simulink model "I2C_V2"  (R2017b)
settings: Solver=FixedStepAuto  StartTime=0.0  StopTime=10.0  RelTol=1e-3
PreLoadFcn:
  | waijung.modelPreload; % Required for working with Waijung Blockset. Do not remove.
undefined symbols (not defined in the file): HSEOSC, Link, LQFP100, ST, STM32F407VG
libraries: simulink x51, stm32f4_i2c_lib x7, stm32f4_io_lib x2, stm32f4_device_config_lib x1
(part 1 of 2)
CloseFcn:
  | waijung.modelClose; % Required for working with Waijung Blockset. Do not remove.
settings Model: Creator=Sputnik  LastModifiedBy=Sputnik
settings OptimizationCC: DefaultParameterBehavior=Inlined  PassReuseOutputArgsAs=Individual arguments
settings DebuggingCC: ParameterTunabilityLossMsg=error
settings HardwareCC: ProdBitPerPointer=32  ProdBitPerSizeT=32  ProdBitPerPtrDiffT=32  ProdLargestAtomicFloat=None  ProdIntDivRoundTo=Undefined  ProdWordSize=32  ProdHWDeviceType=ARM Compatible->Cortex - M4  TargetEndianess=LittleEndian  TargetHWDeviceType=ARM Compatible->Cortex - M4
settings SFSimCC: MATLABDynamicMemAlloc=off
settings RTWCC: SystemTargetFile=stm32f4.tlc  GenerateMakefile=off  TemplateMakefile=ert_default_tmf  Description=STM32F4 Target  GenerateReport=on  IncludeHyperlinkInReport=on  LaunchReport=on  GenerateTraceInfo=on  GenerateTraceReport=on  GenerateTraceReportSl=on  GenerateTraceReportSf=on  GenerateTraceReportEml=on
settings CodeAppCC: ForceParamTrailComments=on  IgnoreCustomStorageClasses=off  OperatorAnnotations=on  SimulinkDataObjDesc=on  SFDataObjDesc=on  InsertBlockDesc=on
settings STFCustomTargetCC: TargetLangStandard=C99 (ISO)  MultiwordLength=256  ModelReferenceCompliant=off  CombineOutputUpdateFcns=on  ERTCustomFileBanners=on  SupportContinuousTime=off  SupportNonInlinedSFcns=off  RemoveResetFunc=on  MATLABClassNameForMDSCustomization=Simulink.SoftwareTarget.ERTCustomization  GRTInterface=off  SystemTargetFile=stm32f4.tlc
settings ERTTargetCC: TargetLangStandard=C99 (ISO)  ModelReferenceCompliant=off  ParMdlRefBuildCompliant=off  CompOptLevelCompliant=off  ConcurrentExecutionCompliant=off  ModelStepFunctionPrototypeControlCompliant=off  CPPClassGenCompliant=off  UseToolchainInfoCompliant=off  InlinedParameterPlacement=NonHierarchical  ERTSrcFileBannerTemplate=stm32f4_code_template.cgt  ERTHdrFileBannerTemplate=stm32f4_code_template.cgt  ERTDataSrcFileTemplate=stm32f4_code_template.cgt  ERTDataHdrFileTemplate=stm32f4_code_template.cgt  ERTCustomFileTemplate=stm32f4_file_process.tlc

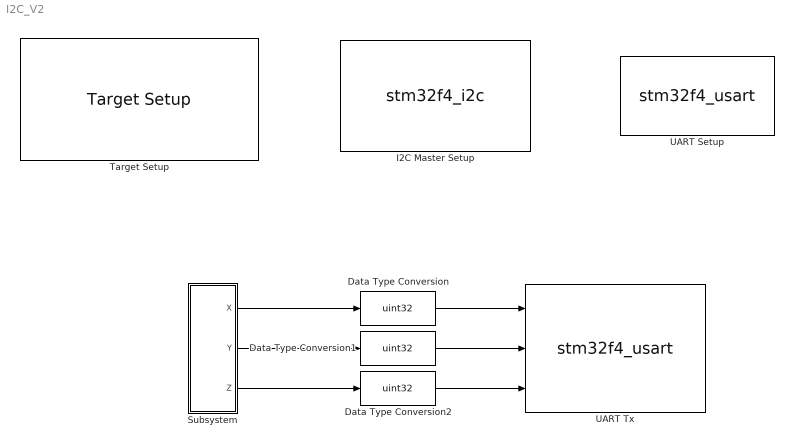
== system I2C_V2 ==
  Data Type Conversion : DataTypeConversion  OutDataTypeStr=uint32
  Data Type Conversion1 : DataTypeConversion  OutDataTypeStr=uint32
  Data Type Conversion2 : DataTypeConversion  OutDataTypeStr=uint32
  I2C Master Setup : S-Function  FunctionName=stm32f4_i2c  Parameters=configuration,module,transfer,clkspeed,timeout,sdapin,sclpin,writecount,readcount,inputtypearray,outputtypearray,confstr,sampletime,sampletimestr,blockid  SFunctionDeploymentMode=off  EnableBusSupport=off  mask(stm32f4_i2c){configuration=Setup, module=1, lastmodule=1, transfer=Blocking, dutycycle=TLow/THigh = 2, clkspeed=400, timeout=25, writecount=0, readcount=0, sdapin=B7, sclpin=B6, waitwritetime=0, inputtypearray=[0], outputtypearray=[0], confstr=["B","7","B","6","1","1","6","0","I2C_DutyCycle_2","0","off"], sampletime=-1, sampletimestr=-1, blockid=I2CMasterSetup}
      mask prompts: module "I2C Module"; lastmodule "Last module"; transfer "Transfer mode"; dutycycle "Duty cycle in fast mode"; clkspeed "Clock speed (kHz)"; timeout "Timeout (ms)"; writecount "Bytes write count"; readcount "Bytes read count"; sdapin "SDA pin"; sclpin "SCL pin"; waitwritetime "Wait write time (ms), default is 0"; inputtypearray "Input type array"; outputtypearray "Output type array"; confstr "Configuration string"; sampletime "Sample time (sec)"; sampletimestr "Compiled sample time (sec) in string"
      mask init:
      | stm32f4_i2c_callback('init');
      mask Help: web(fullfile(waijungdocroot,'stm32f4_i2c_setup.htm'), '-browser')
      mask TypeOptions configuration: Setup | Transaction
      mask Callback configuration: stm32f4_i2c_callback('configuration');
      mask TypeOptions module: 1 | 2 | 3
      mask Callback module: stm32f4_i2c_callback('module');
      mask TypeOptions transfer: Blocking | Non-blocking
      mask TypeOptions dutycycle: TLow/THigh = 16/9 | TLow/THigh = 2
      mask Callback dutycycle: stm32f4_i2c_callback('dutycycle');
      mask Callback writecount: stm32f4_i2c_callback('writecount');
      mask Callback readcount: stm32f4_i2c_callback('readcount');
      mask TypeOptions sdapin: Not used | B7 | B9
      mask Callback sdapin: stm32f4_i2c_callback('sdapin');
      mask TypeOptions sclpin: Not used | B6 | B8
      mask Callback sclpin: stm32f4_i2c_callback('sclpin');
      mask Callback confstr: stm32f4_i2c_callback('confstr');
      mask Callback sampletime: stm32f4_i2c_callback('sampletime');
      mask Callback sampletimestr: stm32f4_i2c_callback('sampletimestr');
      mask Callback blockid: stm32f4_i2c_callback('blockid');
      mask Display: text(0.5, 0.5, 'Module: I2C1\nClock: 400kHz\nSDA/SCL Pin: B7/B6','ver','middle','hor','center');
  Subsystem : Subsystem
  Target Setup : stm32f4_device_config_lib/Target Setup  Priority=100  compiler=GNU ARM  previous_compiler=GNU ARM  mcu=STM32F407VG (LQFP100)  mcustr=STM32F407VG  clockconfig=HSEOSC-8MHz  system_stm32f4xx_c_path=C:\Users\Sputnik\Downloads\waijung17_03a\targets\stm32f4_target\stm32f4\utils\system_stm32f4xx_default\STM32F40_41xxx\hseosc8mhz  showmemoryconfiguration=off  stacksize=0x2000  heapsize=0x2000  enableautocompiledownload=on  fullchiperase=off  programmerinterface=ST-Link  editctrlstr=on  compilercontrolstr=$(patsubst %, -I%, .) -mcpu=cortex-m4 -mthumb -mthumb-interwork -mfloat-abi=hard -mfpu=fpv4-sp-d16 -ffast-math -Wall -Wextra -Ofast  assemblercontrolstr=$(patsubst %, -I%, .) -mcpu=cortex-m4 -mthumb -mthumb-interwork -mfloat-abi=hard -mfpu=fpv4-sp-d16 -ffast-math -Wall -Wextra -Ofast -Wa,-amhls=$(<:.s=.lst) -D__STACK_SIZE=$(STACK_SIZE) -D__HEAP_SIZE=$(HEAP_SIZE)  linkercontrolstr=-T$(LD_SCRIPT) -g -Wl,-Map=$(MAP),--cref,--no-warn-mismatch -mcpu=cortex-m4 -mthumb -mthumb-interwork -mfloat-abi=hard -mfpu=fpv4-sp-d16  runafterdownload=on  execprofile=None  profileruart=3  profilerbaud=500000  profilertxpin=D8  profilerinitstr=0.005,168000000,840000,500000,0  manualsetsampletime=on  sampletime=0.005  blockid=TargetSetup  systickreloadvalue=840000  hseval=8000000  lastprofileruart=3  hclk=168000000  flashorigin=0x8000000  flashlength=1024k  ramorigin=0x20000000  ramlength=128k  useextram=off
      settings: SourceProductName=Waijung Blockset
  UART Setup : S-Function  Priority=1  FunctionName=stm32f4_usart  Parameters=configuration,uartmodule,transfer,baudrate,inputtype,outputtype,confstr,binheaderarray,binterminatorarray,asciiheader,asciiterminator,bindatalength,packetmode,varname,sampletime,sampletimestr,blockid  SFunctionDeploymentMode=off  EnableBusSupport=off  mask(stm32f4_usart){configuration=Setup, uartmodule=4, baudrate=9600, databits=8, parity=No, stopbit=1, remaptxpin=C10, remaprxpin=C11, flowcontrol=None, remapctspin=Not used, remaprtspin=Not used, advanceoptions=on, rxbuffersize=512, txbuffersize=512, transfer=Blocking, packetmode=Ascii, binheader='7E 7E', binterminator='03 03', porttype_double=1, porttype_single=0, porttype_int8=1, porttype_uint8=0, porttype_int16=0, porttype_uint16=0, porttype_int32=0, porttype_uint32=0, asciiformat='%d,%f', rx_asciiterminator=CRLF (0x0D 0x0A - "\r\n"), tx_asciiterminator=CR (0x0D - "\r"), storagename=<empty>, varname=, inputtype=[0], outputtype=[0], binheaderarray=[0], binterminatorarray=[0], bindatalength=0, asciiheader='', asciiterminator=[0], sampletime=-1, sampletimestr=-1, blockid=UARTSetup, confstr=[ "dummy", "1", "C", "10", "1", "C", "11", "0", "*", "*", "0", "*", "*", "1", "4", "4", "1", "4", "2", "512", "512", "1", "4", "9600", "8", "No", "1", "None", "UART4"], lastmodule=4}
      mask prompts: uartmodule "UART Module"; baudrate "Baud rate (bps)"; databits "Data bits"; stopbit "Stop bit"; remaptxpin "Tx Pin"; remaprxpin "Rx Pin"; flowcontrol "Hardware flow control"; remapctspin "HW Flow control, CTS Pin"; remaprtspin "HW Flow control, RTS Pin"; advanceoptions "Advance options"; rxbuffersize "Rx buffer size (bytes)"; txbuffersize "Tx buffer size (bytes)"; packetmode "Packet mode"; binheader "Binary header (example: '7E 7E')"; binterminator "Binary terminator (example: '03 03')"; porttype_double "Number of data port, type DOUBLE"; porttype_single "Number of data port, type SINGLE"; porttype_int8 "Number of data port, type INT8"; porttype_uint8 "Number of data port, type UINT8"; porttype_int16 "Number of data port, type INT16"; porttype_uint16 "Number of data port, type UINT16"; porttype_int32 "Number of data port, type INT32"; porttype_uint32 "Number of data port, type UINT32"; asciiformat "Ascii format"; rx_asciiterminator "End of packet"; tx_asciiterminator "End of packet"; storagename "Buffer"; varname "Var name"; inputtype "Input data type"; outputtype "Output data type"; binheaderarray "Binary header"; binterminatorarray "Binary terminator"; bindatalength "Binary data length"; asciiheader "Ascii header (printf format)"; asciiterminator "Ascii terminator"; sampletime "Sample time (sec)"; sampletimestr "Compiled sample time (sec) in string"; confstr "Configuration string"; lastmodule "Last module selected"
      mask help:
      | Default STM32F4DISCOVERY + aMG F4 Connect 2 + aMG USB Converter N2 settings use
      |
      | USART3, Tx D8, Rx D9 and USB Serial Converter A.
      mask init:
      | stm32f4_usart_callback('init');
      mask Help: web(fullfile(waijungdocroot,'stm32f4_usart_setup.htm'), '-browser')
      mask TypeOptions configuration: Setup | Tx | Rx
      mask Callback configuration: stm32f4_usart_callback('configuration');
      mask TypeOptions uartmodule: 1 | 2 | 3 | 4 | 5 | 6
      mask Callback uartmodule: stm32f4_usart_callback('uartmodule');
      mask Callback baudrate: stm32f4_usart_callback('baudrate');
      mask TypeOptions databits: 8
      mask TypeOptions parity: No | Odd | Even
      mask TypeOptions stopbit: 0.5 | 1 | 1.5 | 2
      mask TypeOptions remaptxpin: Not used | A0 | C10
      mask TypeOptions remaprxpin: Not used | A1 | C11
      mask TypeOptions flowcontrol: None | RTS | CTS | RTS/CTS
      mask Callback flowcontrol: stm32f4_usart_callback('flowcontrol');
      mask TypeOptions remapctspin: Not used
      mask TypeOptions remaprtspin: Not used
      mask Callback advanceoptions: stm32f4_usart_callback('advanceoptions');
      mask TypeOptions rxbuffersize: 16 | 32 | 64 | 128 | 256 | 512 | 1024 | 2048
      mask TypeOptions txbuffersize: 16 | 32 | 64 | 128 | 256 | 512 | 1024 | 2048
      mask TypeOptions transfer: Blocking | Non-Blocking
      mask Callback transfer: stm32f4_usart_callback('transfer');
      mask TypeOptions packetmode: Ascii | Binary | String Buffer
      mask Callback packetmode: stm32f4_usart_callback('packetmode');
      mask Callback binheader: stm32f4_usart_callback('binheader');
      mask Callback binterminator: stm32f4_usart_callback('binterminator');
      mask Callback porttype_double: stm32f4_usart_callback('porttype');
      mask Callback porttype_single: stm32f4_usart_callback('porttype');
      mask Callback porttype_int8: stm32f4_usart_callback('porttype');
      mask Callback porttype_uint8: stm32f4_usart_callback('porttype');
      mask Callback porttype_int16: stm32f4_usart_callback('porttype');
      mask Callback porttype_uint16: stm32f4_usart_callback('porttype');
      mask Callback porttype_int32: stm32f4_usart_callback('porttype');
      mask Callback porttype_uint32: stm32f4_usart_callback('porttype');
      mask Callback asciiformat: stm32f4_usart_callback('asciiformat');
      mask TypeOptions rx_asciiterminator: CR (0x0D - "\r") | LF (0x0A - "\n") | CRLF (0x0D 0x0A - "\r\n")
      mask Callback rx_asciiterminator: stm32f4_usart_callback('rx_asciiterminator');
      mask TypeOptions tx_asciiterminator: CR (0x0D - "\r") | LF (0x0A - "\n") | CRLF (0x0D 0x0A - "\r\n") | None
      mask Callback tx_asciiterminator: stm32f4_usart_callback('tx_asciiterminator');
      mask TypeOptions storagename: <empty>
      mask Callback storagename: stm32f4_usart_callback('storagename');
      mask Callback varname: stm32f4_usart_callback('varname');
      mask Callback sampletime: stm32f4_usart_callback('sampletime');
      mask Callback sampletimestr: stm32f4_usart_callback('sampletimestr');
      mask Callback blockid: stm32f4_usart_callback('blockid');
      mask Display: text(0.5, 0.5, 'Module: UART4_Setup\nBaud (Bps): 9600\nDMA Buffer: 512/512\nTx/Rx Pin: C10/C11','ver','middle','hor','center');
  UART Tx : S-Function  Priority=1  FunctionName=stm32f4_usart  Parameters=configuration,uartmodule,transfer,baudrate,inputtype,outputtype,confstr,binheaderarray,binterminatorarray,asciiheader,asciiterminator,bindatalength,packetmode,varname,sampletime,sampletimestr,blockid  SFunctionDeploymentMode=off  EnableBusSupport=off  mask(stm32f4_usart){configuration=Tx, uartmodule=4, baudrate=115200, databits=8, parity=No, stopbit=1, remaptxpin=Not used, remaprxpin=Not used, flowcontrol=None, remapctspin=Not used, remaprtspin=Not used, advanceoptions=off, rxbuffersize=512, txbuffersize=512, transfer=Non-Blocking, packetmode=Ascii, binheader='', binterminator='', porttype_double=0, porttype_single=0, porttype_int8=0, porttype_uint8=0, porttype_int16=0, porttype_uint16=3, porttype_int32=0, porttype_uint32=0, asciiformat='value=%u,%u,%u', rx_asciiterminator=CRLF (0x0D 0x0A - "\r\n"), tx_asciiterminator=CRLF (0x0D 0x0A - "\r\n"), storagename=<empty>, varname=, inputtype=[3  7 7 7], outputtype=[0], binheaderarray=[0], binterminatorarray=[0], bindatalength=0, asciiheader='value=%u,%u,%u\r\n', asciiterminator=[2 13 10], sampletime=0.005, sampletimestr=-1, blockid=UARTTx, confstr=[ "dummy", "0", "*", "*", "0", "*", "*", "0", "*", "*", "0", "*", "*", "1", "4", "4", "1", "4", "2", "512", "512", "1", "4", "115200", "8", "No", "1", "None", "UART4"], lastmodule=1}
      mask prompts: uartmodule "UART Module"; baudrate "Baud rate (bps)"; databits "Data bits"; stopbit "Stop bit"; remaptxpin "Tx Pin"; remaprxpin "Rx Pin"; flowcontrol "Hardware flow control"; remapctspin "HW Flow control, CTS Pin"; remaprtspin "HW Flow control, RTS Pin"; advanceoptions "Advance options"; rxbuffersize "Rx buffer size (bytes)"; txbuffersize "Tx buffer size (bytes)"; packetmode "Packet mode"; binheader "Binary header (example: '7E 7E')"; binterminator "Binary terminator (example: '03 03')"; porttype_double "Number of data port, type DOUBLE"; porttype_single "Number of data port, type SINGLE"; porttype_int8 "Number of data port, type INT8"; porttype_uint8 "Number of data port, type UINT8"; porttype_int16 "Number of data port, type INT16"; porttype_uint16 "Number of data port, type UINT16"; porttype_int32 "Number of data port, type INT32"; porttype_uint32 "Number of data port, type UINT32"; asciiformat "Ascii format"; rx_asciiterminator "End of packet"; tx_asciiterminator "End of packet"; storagename "Buffer"; varname "Var name"; inputtype "Input data type"; outputtype "Output data type"; binheaderarray "Binary header"; binterminatorarray "Binary terminator"; bindatalength "Binary data length"; asciiheader "Ascii header (printf format)"; asciiterminator "Ascii terminator"; sampletime "Sample time (sec)"; sampletimestr "Compiled sample time (sec) in string"; confstr "Configuration string"; lastmodule "Last module selected"
      mask help:
      | Data type for Ascii format
      | %u, %i, %d, %o, %x: uint32
      | %e, %g, %f: single
      | %c: int8
      mask init:
      | stm32f4_usart_callback('init');
      mask Help: web(fullfile(waijungdocroot,'stm32f4_usart_tx.htm'), '-browser')
      mask TypeOptions configuration: Setup | Tx | Rx
      mask Callback configuration: stm32f4_usart_callback('configuration');
      mask TypeOptions uartmodule: 1 | 2 | 3 | 4 | 5 | 6
      mask Callback uartmodule: stm32f4_usart_callback('uartmodule');
      mask Callback baudrate: stm32f4_usart_callback('baudrate');
      mask TypeOptions databits: 8
      mask TypeOptions parity: No | Odd | Even
      mask TypeOptions stopbit: 0.5 | 1 | 1.5 | 2
      mask TypeOptions remaptxpin: Not used | A9 | B6
      mask TypeOptions remaprxpin: Not used | A10 | B7
      mask TypeOptions flowcontrol: None | RTS | CTS | RTS/CTS
      mask Callback flowcontrol: stm32f4_usart_callback('flowcontrol');
      mask TypeOptions remapctspin: Not used | A11
      mask TypeOptions remaprtspin: Not used | A12
      mask Callback advanceoptions: stm32f4_usart_callback('advanceoptions');
      mask TypeOptions rxbuffersize: 16 | 32 | 64 | 128 | 256 | 512 | 1024 | 2048
      mask TypeOptions txbuffersize: 16 | 32 | 64 | 128 | 256 | 512 | 1024 | 2048
      mask TypeOptions transfer: Blocking | Non-Blocking
      mask Callback transfer: stm32f4_usart_callback('transfer');
      mask TypeOptions packetmode: Ascii | Binary | Binary Vector | String Buffer
      mask Callback packetmode: stm32f4_usart_callback('packetmode');
      mask Callback binheader: stm32f4_usart_callback('binheader');
      mask Callback binterminator: stm32f4_usart_callback('binterminator');
      mask Callback porttype_double: stm32f4_usart_callback('porttype');
      mask Callback porttype_single: stm32f4_usart_callback('porttype');
      mask Callback porttype_int8: stm32f4_usart_callback('porttype');
      mask Callback porttype_uint8: stm32f4_usart_callback('porttype');
      mask Callback porttype_int16: stm32f4_usart_callback('porttype');
      mask Callback porttype_uint16: stm32f4_usart_callback('porttype');
      mask Callback porttype_int32: stm32f4_usart_callback('porttype');
      mask Callback porttype_uint32: stm32f4_usart_callback('porttype');
      mask Callback asciiformat: stm32f4_usart_callback('asciiformat');
      mask TypeOptions rx_asciiterminator: CR (0x0D - "\r") | LF (0x0A - "\n") | CRLF (0x0D 0x0A - "\r\n")
      mask Callback rx_asciiterminator: stm32f4_usart_callback('rx_asciiterminator');
      mask TypeOptions tx_asciiterminator: CR (0x0D - "\r") | LF (0x0A - "\n") | CRLF (0x0D 0x0A - "\r\n") | None
      mask Callback tx_asciiterminator: stm32f4_usart_callback('tx_asciiterminator');
      mask TypeOptions storagename: <empty>
      mask Callback storagename: stm32f4_usart_callback('storagename');
      mask Callback varname: stm32f4_usart_callback('varname');
      mask Callback sampletime: stm32f4_usart_callback('sampletime');
      mask Callback sampletimestr: stm32f4_usart_callback('sampletimestr');
      mask Callback blockid: stm32f4_usart_callback('blockid');
      mask Display: text(0.5, 0.5, 'Module: UART4_Tx\nPacket: Ascii\nTransfer: Non-Blocking\nTs (sec): -1','ver','middle','hor','center'); port_label('input', 1,'uint32'); port_label('input', 2,'uint32'); port_label('input', 3,'uint32');
  wires:
  Data Type Conversion/1 -> UART Tx/1
  Data Type Conversion1/1 -> UART Tx/2
  Data Type Conversion2/1 -> UART Tx/3
  Subsystem/1(X) -> Data Type Conversion/1
  Subsystem/2(Y) -> Data Type Conversion1/1
  Subsystem/3(Z) -> Data Type Conversion2/1

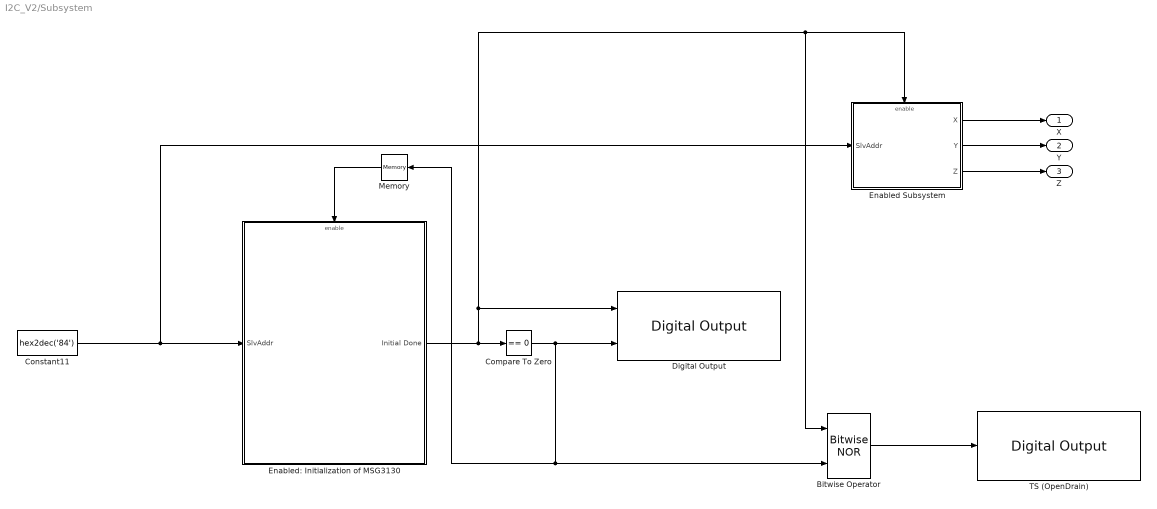
== system I2C_V2/Subsystem ==
  Bitwise Operator : simulink/Logic and Bit Operations/Bitwise Operator  logicop=NOR  UseBitMask=off  NumInputPorts=2  BitMask=bin2dec('11011001')  BitMaskRealWorld=Stored Integer
  Compare To Zero : simulink/Logic and Bit Operations/Compare To Zero  relop===  OutDataTypeStr=boolean  ZeroCross=off
  Constant11 : Constant  Value=hex2dec('84')  OutDataTypeStr=uint8  SampleTime=0.5
  Digital Output : stm32f4_io_lib/Digital Output  use_bitband=on  port=D  speed=100  porttype=Push Pull  porttypestr=PP  use_pin0=off  use_pin1=off  use_pin2=off  use_pin3=off  use_pin4=off  use_pin5=off  use_pin6=off  use_pin7=off  use_pin8=off  use_pin9=off  use_pin10=off  use_pin11=off  use_pin12=on  use_pin13=off  use_pin14=on  use_pin15=off  pinstr=GPIO_Pin_12 | GPIO_Pin_14  usedpinarray="[0  0  0  0  0  0  0  0  0  0  0  0  1  0  1  0]"  bitbandingstr=|  sampletime=-1  sampletimestr=-1  blockid=SubsystemDigitalOutput  enablecustomportlabel=off  globalinit=off  cinputportlabel=In1, In2  coutputportlabel=0
      | #define SubsystemDigitalOutput_D12 Peripheral_BB(GPIOD->ODR, 12)  /* Output pin */
      | #define SubsystemDigitalOutput_D14 Peripheral_BB(GPIOD->ODR, 14)  /* Output pin */
  Enabled Subsystem : Subsystem  TreatAsAtomicUnit=on
  Enabled: Initialization of MSG3130 : Subsystem  TreatAsAtomicUnit=on
  Memory : Memory  InheritSampleTime=on
  TS (OpenDrain) : stm32f4_io_lib/Digital Output  use_bitband=on  port=A  speed=100  porttype=Open Drain  porttypestr=OD  use_pin0=off  use_pin1=off  use_pin2=off  use_pin3=off  use_pin4=off  use_pin5=off  use_pin6=off  use_pin7=off  use_pin8=off  use_pin9=off  use_pin10=off  use_pin11=off  use_pin12=off  use_pin13=off  use_pin14=off  use_pin15=on  pinstr=GPIO_Pin_15  usedpinarray="[0  0  0  0  0  0  0  0  0  0  0  0  0  0  0  1]"  bitbandingstr="#define SubsystemTSOpenDrain_A15 Peripheral_BB(GPIOA->ODR, 15)  /* Output pin */"  sampletime=-1  sampletimestr=-1  blockid=SubsystemTSOpenDrain  enablecustomportlabel=off  globalinit=off  cinputportlabel=In1, In2  coutputportlabel=0
  X : Outport
  Y : Outport  Port=2
  Z : Outport  Port=3
  wires:
  Compare To Zero/1 -> Digital Output/2, Memory/1, Bitwise Operator/2
  Enabled: Initialization of MSG3130/1(Initial Done) -> Digital Output/1, Bitwise Operator/1, Enabled Subsystem/Enable, Compare To Zero/1
  Constant11/1 -> Enabled Subsystem/1(SlvAddr), Enabled: Initialization of MSG3130/1(SlvAddr)
  Bitwise Operator/1 -> TS (OpenDrain)/1
  Memory/1 -> Enabled: Initialization of MSG3130/Enable
  Enabled Subsystem/1(X) -> X/1
  Enabled Subsystem/2(Y) -> Y/1
  Enabled Subsystem/3(Z) -> Z/1

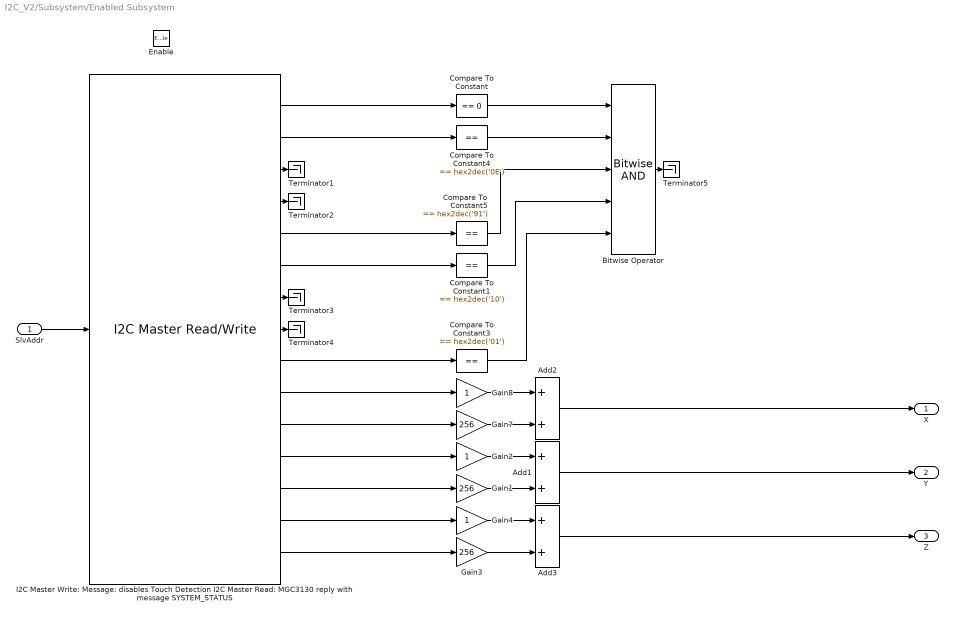
== system I2C_V2/Subsystem/Enabled Subsystem ==
  SlvAddr : Inport
  Enable : EnablePort
  Add1 : Sum  AccumDataTypeStr=int16
  Add2 : Sum  AccumDataTypeStr=int16
  Add3 : Sum  AccumDataTypeStr=int16
  Bitwise Operator : simulink/Logic and Bit Operations/Bitwise Operator  logicop=AND  UseBitMask=off  NumInputPorts=5  BitMask=bin2dec('11011001')  BitMaskRealWorld=Stored Integer
  Compare To Constant : simulink/Logic and Bit Operations/Compare To Constant  relop===  const=0  OutDataTypeStr=boolean  ZeroCross=off
  Compare To Constant1 : simulink/Logic and Bit Operations/Compare To Constant  relop===  const=hex2dec('10')  OutDataTypeStr=boolean  ZeroCross=off
  Compare To Constant3 : simulink/Logic and Bit Operations/Compare To Constant  relop===  const=hex2dec('01')  OutDataTypeStr=boolean  ZeroCross=off
  Compare To Constant4 : simulink/Logic and Bit Operations/Compare To Constant  relop===  const=hex2dec('0E')  OutDataTypeStr=boolean  ZeroCross=off
  Compare To Constant5 : simulink/Logic and Bit Operations/Compare To Constant  relop===  const=hex2dec('91')  OutDataTypeStr=boolean  ZeroCross=off
  Gain1 : Gain  Gain=256  OutDataTypeStr=uint16
  Gain2 : Gain  OutDataTypeStr=uint16
  Gain3 : Gain  Gain=256  OutDataTypeStr=uint16
  Gain4 : Gain  OutDataTypeStr=uint16
  Gain7 : Gain  Gain=256  OutDataTypeStr=uint16
  Gain8 : Gain  OutDataTypeStr=uint16
  "I2C Master Write: Message: disables Touch Detection I2C Master Read: MGC3130 reply with message SYSTEM_STATUS " : stm32f4_i2c_lib/I2C Master Read//Write  configuration=Transaction  module=1  lastmodule=3  transfer=Blocking  dutycycle=TLow/THigh = 2  clkspeed=400  timeout=25  writecount=0  readcount=14  sdapin=C9  sclpin=A8  waitwritetime=1  forcestop=on  inputtypearray=[1 3]  outputtypearray=[15 3 3 3 3 3 3 3 3 3 3 3 3 3 3 3]  confstr="[\"C\",\"9\",\"A\",\"8\",\"1\",\"1\",\"6\",\"0\",\"I2C_DutyCycle_2\",\"1\",\"on\"]"  sampletime=0.01  sampletimestr=-1  blockid=SubsystemEnabledSubsystemI2CMasterWriteMessagedisablesTouchDetectionI2CMasterReadMGC3130replywithmessageSYSTEM_STATUS
  Terminator{1..5} (5 alike) : Terminator
  X : Outport
  Y : Outport  Port=2
  Z : Outport  Port=3
  wires:
  SlvAddr/1 -> "I2C Master Write: Message: disables Touch Detection I2C Master Read: MGC3130 reply with message SYSTEM_STATUS "/1
  "I2C Master Write: Message: disables Touch Detection I2C Master Read: MGC3130 reply with message SYSTEM_STATUS "/1 -> Compare To Constant/1
  "I2C Master Write: Message: disables Touch Detection I2C Master Read: MGC3130 reply with message SYSTEM_STATUS "/2 -> Compare To Constant4/1
  "I2C Master Write: Message: disables Touch Detection I2C Master Read: MGC3130 reply with message SYSTEM_STATUS "/3 -> Terminator1/1
  "I2C Master Write: Message: disables Touch Detection I2C Master Read: MGC3130 reply with message SYSTEM_STATUS "/4 -> Terminator2/1
  "I2C Master Write: Message: disables Touch Detection I2C Master Read: MGC3130 reply with message SYSTEM_STATUS "/5 -> Compare To Constant5/1
  "I2C Master Write: Message: disables Touch Detection I2C Master Read: MGC3130 reply with message SYSTEM_STATUS "/6 -> Compare To Constant1/1
  "I2C Master Write: Message: disables Touch Detection I2C Master Read: MGC3130 reply with message SYSTEM_STATUS "/7 -> Terminator3/1
  "I2C Master Write: Message: disables Touch Detection I2C Master Read: MGC3130 reply with message SYSTEM_STATUS "/8 -> Terminator4/1
  "I2C Master Write: Message: disables Touch Detection I2C Master Read: MGC3130 reply with message SYSTEM_STATUS "/9 -> Compare To Constant3/1
  Compare To Constant/1 -> Bitwise Operator/1
  Compare To Constant4/1 -> Bitwise Operator/2
  Compare To Constant5/1 -> Bitwise Operator/3
  Compare To Constant1/1 -> Bitwise Operator/4
  Compare To Constant3/1 -> Bitwise Operator/5
  "I2C Master Write: Message: disables Touch Detection I2C Master Read: MGC3130 reply with message SYSTEM_STATUS "/10 -> Gain8/1
  "I2C Master Write: Message: disables Touch Detection I2C Master Read: MGC3130 reply with message SYSTEM_STATUS "/11 -> Gain7/1
  Gain8/1 -> Add2/1
  Gain7/1 -> Add2/2
  Gain2/1 -> Add1/1
  Gain1/1 -> Add1/2
  "I2C Master Write: Message: disables Touch Detection I2C Master Read: MGC3130 reply with message SYSTEM_STATUS "/12 -> Gain2/1
  "I2C Master Write: Message: disables Touch Detection I2C Master Read: MGC3130 reply with message SYSTEM_STATUS "/13 -> Gain1/1
  Gain4/1 -> Add3/1
  Gain3/1 -> Add3/2
  "I2C Master Write: Message: disables Touch Detection I2C Master Read: MGC3130 reply with message SYSTEM_STATUS "/14 -> Gain4/1
  "I2C Master Write: Message: disables Touch Detection I2C Master Read: MGC3130 reply with message SYSTEM_STATUS "/15 -> Gain3/1
  Add2/1 -> X/1
  Add1/1 -> Y/1
  Add3/1 -> Z/1
  Bitwise Operator/1 -> Terminator5/1

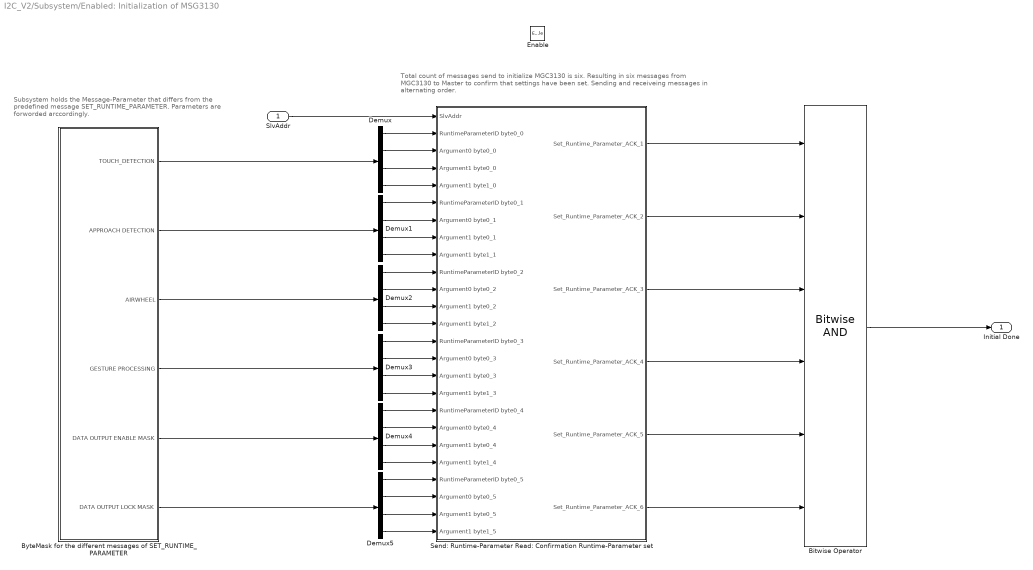
== system I2C_V2/Subsystem/Enabled: Initialization of MSG3130 ==
  note: Subsystem holds the Message-Parameter that differs
      | from the predefined message SET_RUNTIME_PARAMETER.
      | Parameters are forworded arccordingly.
  note: Total count of messages send to initialize MGC3130 is six.
      | Resulting in six messages from MGC3130 to Master to confirm that settings have been set.
      | Sending and receiveing messages in alternating order.
  SlvAddr : Inport
  Enable : EnablePort
  Bitwise Operator : simulink/Logic and Bit Operations/Bitwise Operator  logicop=AND  UseBitMask=off  NumInputPorts=6  BitMask=bin2dec('11011001')  BitMaskRealWorld=Stored Integer
  ByteMask for the different messages of SET_RUNTIME_PARAMETER : Subsystem
  Demux{,1..5} (6 alike) : Demux
  Send: Runtime-Parameter Read: Confirmation Runtime-Parameter set : Subsystem
  Initial Done : Outport
  wires:
  ByteMask for the different messages of SET_RUNTIME_PARAMETER/1(TOUCH_DETECTION) -> Demux/1
  ByteMask for the different messages of SET_RUNTIME_PARAMETER/2(APPROACH DETECTION) -> Demux1/1
  ByteMask for the different messages of SET_RUNTIME_PARAMETER/3(AIRWHEEL) -> Demux2/1
  ByteMask for the different messages of SET_RUNTIME_PARAMETER/4(GESTURE PROCESSING) -> Demux3/1
  ByteMask for the different messages of SET_RUNTIME_PARAMETER/5(DATA OUTPUT ENABLE MASK) -> Demux4/1
  ByteMask for the different messages of SET_RUNTIME_PARAMETER/6(DATA OUTPUT LOCK MASK) -> Demux5/1
  Demux/1 -> Send: Runtime-Parameter Read: Confirmation Runtime-Parameter set/2(RuntimeParameterID byte0_0)
  Demux/2 -> Send: Runtime-Parameter Read: Confirmation Runtime-Parameter set/3(Argument0 byte0_0)
  Demux/3 -> Send: Runtime-Parameter Read: Confirmation Runtime-Parameter set/4(Argument1 byte0_0)
  Demux/4 -> Send: Runtime-Parameter Read: Confirmation Runtime-Parameter set/5(Argument1 byte1_0)
  Demux1/1 -> Send: Runtime-Parameter Read: Confirmation Runtime-Parameter set/6(RuntimeParameterID byte0_1)
  Demux1/2 -> Send: Runtime-Parameter Read: Confirmation Runtime-Parameter set/7(Argument0 byte0_1)
  Demux1/3 -> Send: Runtime-Parameter Read: Confirmation Runtime-Parameter set/8(Argument1 byte0_1)
  Demux1/4 -> Send: Runtime-Parameter Read: Confirmation Runtime-Parameter set/9(Argument1 byte1_1)
  Demux2/1 -> Send: Runtime-Parameter Read: Confirmation Runtime-Parameter set/10(RuntimeParameterID byte0_2)
  Demux2/2 -> Send: Runtime-Parameter Read: Confirmation Runtime-Parameter set/11(Argument0 byte0_2)
  Demux2/3 -> Send: Runtime-Parameter Read: Confirmation Runtime-Parameter set/12(Argument1 byte0_2)
  Demux2/4 -> Send: Runtime-Parameter Read: Confirmation Runtime-Parameter set/13(Argument1 byte1_2)
  Demux3/1 -> Send: Runtime-Parameter Read: Confirmation Runtime-Parameter set/14(RuntimeParameterID byte0_3)
  Demux3/2 -> Send: Runtime-Parameter Read: Confirmation Runtime-Parameter set/15(Argument0 byte0_3)
  Demux3/3 -> Send: Runtime-Parameter Read: Confirmation Runtime-Parameter set/16(Argument1 byte0_3)
  Demux3/4 -> Send: Runtime-Parameter Read: Confirmation Runtime-Parameter set/17(Argument1 byte1_3)
  Demux4/1 -> Send: Runtime-Parameter Read: Confirmation Runtime-Parameter set/18(RuntimeParameterID byte0_4)
  Demux4/2 -> Send: Runtime-Parameter Read: Confirmation Runtime-Parameter set/19(Argument0 byte0_4)
  Demux4/3 -> Send: Runtime-Parameter Read: Confirmation Runtime-Parameter set/20(Argument1 byte0_4)
  Demux4/4 -> Send: Runtime-Parameter Read: Confirmation Runtime-Parameter set/21(Argument1 byte1_4)
  Demux5/1 -> Send: Runtime-Parameter Read: Confirmation Runtime-Parameter set/22(RuntimeParameterID byte0_5)
  Demux5/2 -> Send: Runtime-Parameter Read: Confirmation Runtime-Parameter set/23(Argument0 byte0_5)
  Demux5/3 -> Send: Runtime-Parameter Read: Confirmation Runtime-Parameter set/24(Argument1 byte0_5)
  Demux5/4 -> Send: Runtime-Parameter Read: Confirmation Runtime-Parameter set/25(Argument1 byte1_5)
  Send: Runtime-Parameter Read: Confirmation Runtime-Parameter set/1(Set_Runtime_Parameter_ACK_1) -> Bitwise Operator/1
  Send: Runtime-Parameter Read: Confirmation Runtime-Parameter set/2(Set_Runtime_Parameter_ACK_2) -> Bitwise Operator/2
  Send: Runtime-Parameter Read: Confirmation Runtime-Parameter set/3(Set_Runtime_Parameter_ACK_3) -> Bitwise Operator/3
  Send: Runtime-Parameter Read: Confirmation Runtime-Parameter set/4(Set_Runtime_Parameter_ACK_4) -> Bitwise Operator/4
  Send: Runtime-Parameter Read: Confirmation Runtime-Parameter set/5(Set_Runtime_Parameter_ACK_5) -> Bitwise Operator/5
  Send: Runtime-Parameter Read: Confirmation Runtime-Parameter set/6(Set_Runtime_Parameter_ACK_6) -> Bitwise Operator/6
  SlvAddr/1 -> Send: Runtime-Parameter Read: Confirmation Runtime-Parameter set/1(SlvAddr)
  Bitwise Operator/1 -> Initial Done/1

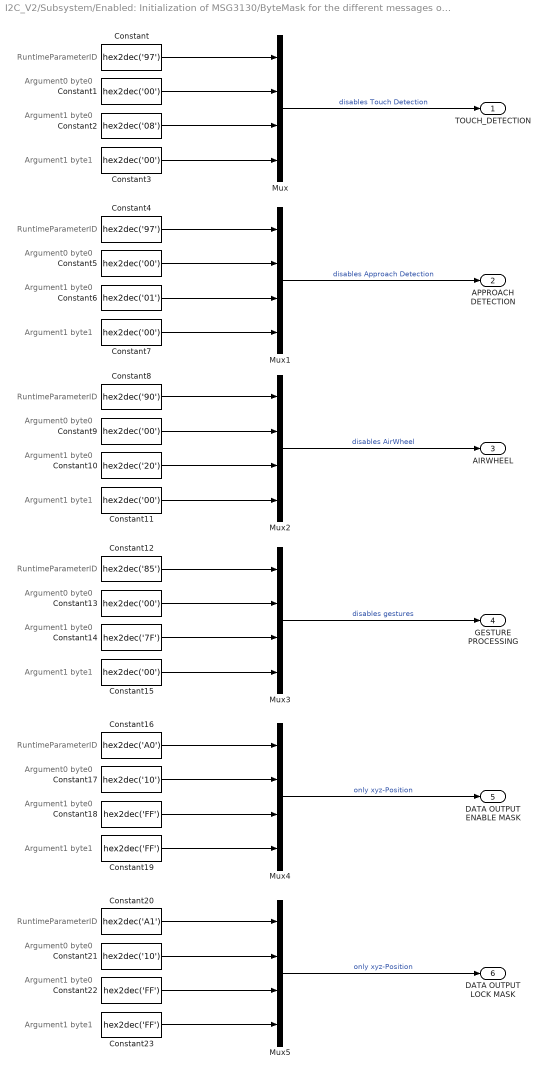
== system I2C_V2/Subsystem/Enabled: Initialization of MSG3130/ByteMask for the different messages of SET_RUNTIME_PARAMETER ==
  note: Argument1 byte0
  note: Argument0 byte0
  note: RuntimeParameterID
  note: Argument1 byte1
  note: RuntimeParameterID
  note: Argument1 byte1
  note: Argument1 byte0
  note: Argument0 byte0
  note: RuntimeParameterID
  note: Argument1 byte1
  note: Argument1 byte0
  note: Argument0 byte0
  note: RuntimeParameterID
  note: Argument1 byte1
  note: Argument1 byte0
  note: Argument0 byte0
  note: RuntimeParameterID
  note: Argument1 byte1
  note: Argument1 byte0
  note: Argument0 byte0
  note: RuntimeParameterID
  note: Argument1 byte1
  note: Argument1 byte0
  note: Argument0 byte0
  Constant : Constant  Value=hex2dec('97')  OutDataTypeStr=uint8
  Constant{1,3,5,7,9,11,13,15} (8 alike) : Constant  Value=hex2dec('00')  OutDataTypeStr=uint8
  Constant10 : Constant  Value=hex2dec('20')  OutDataTypeStr=uint8
  Constant12 : Constant  Value=hex2dec('85')  OutDataTypeStr=uint8
  Constant14 : Constant  Value=hex2dec('7F')  OutDataTypeStr=uint8
  Constant16 : Constant  Value=hex2dec('A0')  OutDataTypeStr=uint8
  Constant17 : Constant  Value=hex2dec('10')  OutDataTypeStr=uint8
  Constant{18..19,22..23} (4 alike) : Constant  Value=hex2dec('FF')  OutDataTypeStr=uint8
  Constant2 : Constant  Value=hex2dec('08')  OutDataTypeStr=uint8
  Constant20 : Constant  Value=hex2dec('A1')  OutDataTypeStr=uint8
  Constant21 : Constant  Value=hex2dec('10')  OutDataTypeStr=uint8
  Constant4 : Constant  Value=hex2dec('97')  OutDataTypeStr=uint8
  Constant6 : Constant  Value=hex2dec('01')  OutDataTypeStr=uint8
  Constant8 : Constant  Value=hex2dec('90')  OutDataTypeStr=uint8
  Mux{,1..5} (6 alike) : Mux
  TOUCH_DETECTION : Outport
  APPROACH DETECTION : Outport  Port=2
  AIRWHEEL : Outport  Port=3
  GESTURE PROCESSING : Outport  Port=4
  DATA OUTPUT ENABLE MASK : Outport  Port=5
  DATA OUTPUT LOCK MASK : Outport  Port=6
  wires:
  Mux/1 -> TOUCH_DETECTION/1  "disables Touch Detection"
  Constant/1 -> Mux/1
  Constant1/1 -> Mux/2
  Constant2/1 -> Mux/3
  Constant3/1 -> Mux/4
  Constant6/1 -> Mux1/3
  Constant7/1 -> Mux1/4
  Constant4/1 -> Mux1/1
  Constant5/1 -> Mux1/2
  Mux1/1 -> APPROACH DETECTION/1  "disables Approach Detection"
  Constant10/1 -> Mux2/3
  Constant11/1 -> Mux2/4
  Constant8/1 -> Mux2/1
  Constant9/1 -> Mux2/2
  Mux2/1 -> AIRWHEEL/1  "disables AirWheel"
  Constant14/1 -> Mux3/3
  Constant15/1 -> Mux3/4
  Constant12/1 -> Mux3/1
  Constant13/1 -> Mux3/2
  Mux3/1 -> GESTURE PROCESSING/1  "disables gestures"
  Constant18/1 -> Mux4/3
  Constant19/1 -> Mux4/4
  Constant16/1 -> Mux4/1
  Constant17/1 -> Mux4/2
  Mux4/1 -> DATA OUTPUT ENABLE MASK/1  "only xyz-Position"
  Constant22/1 -> Mux5/3
  Constant23/1 -> Mux5/4
  Constant20/1 -> Mux5/1
  Constant21/1 -> Mux5/2
  Mux5/1 -> DATA OUTPUT LOCK MASK/1  "only xyz-Position"
